simulink model "P4_sim_LQR"  (R2021b)
settings: Solver=ode45  StartTime=0.0  StopTime=Tmax  RelTol=1e-6  EnableMultiTasking=on
values from neighbouring files (symbols this model uses):
  a = g/L    (= 32.6666666667)    [P4_1.m]    (also in P4_2_1.m; P4_2_2.m; P4_2_3.m; P4_3.m)
  b = k/m    (= 0.1)    [P4_1.m]    (also in P4_2_1.m; P4_2_2.m; P4_2_3.m; P4_3.m)
  c = 1/(m*L^2)    (= 111.111111111)    [P4_1.m]    (also in P4_2_1.m; P4_2_2.m; P4_2_3.m; P4_3.m)
  du_max = 0.15    [P4_1.m]    (also in P4_2_1.m = 100; P4_2_2.m = 100; P4_2_3.m = du_vector(i); P4_3.m = 0.085)
  du_min = -0.15    [P4_1.m]    (also in P4_2_1.m = -100; P4_2_2.m = -100; P4_2_3.m = -du_vector(i); P4_3.m = -0.085)
  h = 0.1    [P4_1.m]    (also in P4_2_1.m; P4_2_2.m; P4_2_3.m; P4_3.m)
  KLQ = dlqr(Apd,Bpd,eye(2),R)    [P4_3.m]
  u_max = 0.15    [P4_1.m]    (also in P4_2_1.m = 100; P4_2_2.m = 100; P4_2_3.m = 100; P4_3.m = 0.22)
  u_min = -0.15    [P4_1.m]    (also in P4_2_1.m = -100; P4_2_2.m = -100; P4_2_3.m = -100; P4_3.m = -0.22)
settings Model: Creator=jomle  LastModifiedBy=User
settings SolverCC: AlgebraicLoopSolver=TrustRegion
settings DataIOCC: LimitDataPoints=on  SaveFormat=Array  ReturnWorkspaceOutputs=off
settings OptimizationCC: LifeSpan=inf
settings DebuggingCC: SFUnexpectedBacktrackingDiag=warning  SFNoUnconditionalDefaultTransitionDiag=warning  SFExecutionAtInitializationDiag=none  SFMachineParentedDataDiag=warning  ArithmeticOperatorsInVariantConditions=warning
settings HardwareCC: ProdBitPerPointer=32  ProdBitPerSizeT=32  ProdBitPerPtrDiffT=32  ProdLargestAtomicFloat=None  ProdIntDivRoundTo=Undefined  ProdEndianess=Unspecified  ProdWordSize=32  ProdHWDeviceType=32-bit Generic
settings ModelReferenceCC: PropagateSignalLabelsOutOfModel=off
settings SFSimCC: SimUseLocalCustomCode=off  CustomCodeUndefinedFunction=UseInterfaceOnly
settings RTWCC: RTWUseLocalCustomCode=off
settings CodeAppCC: StateflowObjectComments=on
settings GRTTargetCC: TargetLangStandard=C89/C90 (ANSI)
settings ConfigComp: CovMetricSettings=dw  CovSaveCumulativeToWorkspaceVar=on  CovSaveSingleToWorkspaceVar=on  CovExternalEMLEnable=off

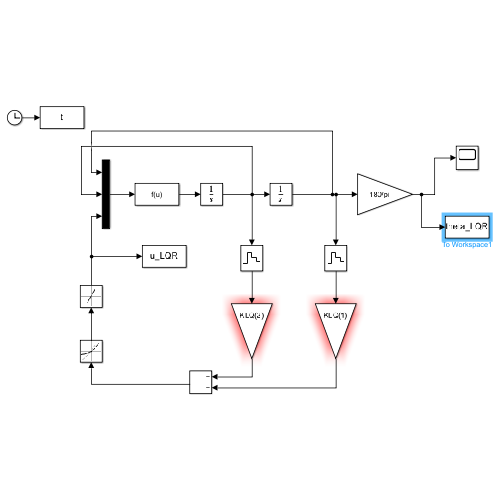
[thumbnail: Simulink's stored preview of the top-level diagram]
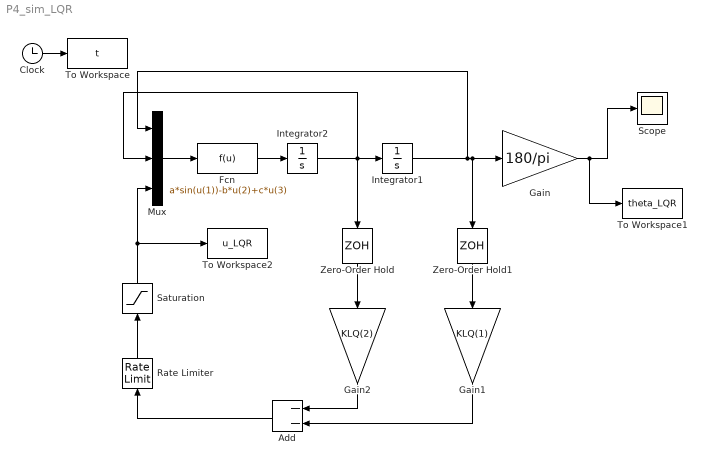
== system P4_sim_LQR ==
  Add : Sum  Inputs=--
  Clock : Clock
  Fcn : Fcn  Expr=a*sin(u(1))-b*u(2)+c*u(3)
  Gain : Gain  Gain=180/pi
  Gain1 : Gain  Gain=KLQ(1)
  Gain2 : Gain  Gain=KLQ(2)
  Integrator1 : Integrator  InitialCondition=30*pi/180
  Integrator2 : Integrator
  Mux : Mux  Inputs=3
  Rate Limiter : RateLimiter  RisingSlewLimit=du_max/h  FallingSlewLimit=du_min/h  SampleTimeMode=inherited
  Saturation : Saturate  UpperLimit=u_max  LowerLimit=u_min
  Scope : Scope
  To Workspace : ToWorkspace  VariableName=t  SampleTime=-1
  To Workspace1 : ToWorkspace  VariableName=theta_LQR  SampleTime=-1
  To Workspace2 : ToWorkspace  VariableName=u_LQR  SaveFormat=Structure With Time  SampleTime=-1
  Zero-Order Hold : ZeroOrderHold  SampleTime=h
  Zero-Order Hold1 : ZeroOrderHold  SampleTime=h
  wires:
  Integrator2/1 -> Mux/2, Zero-Order Hold/1, Integrator1/1
  Integrator1/1 -> Zero-Order Hold1/1, Gain/1, Mux/1
  Gain/1 -> To Workspace1/1, Scope/1
  Mux/1 -> Fcn/1
  Fcn/1 -> Integrator2/1
  Gain2/1 -> Add/1
  Gain1/1 -> Add/2
  Clock/1 -> To Workspace/1
  Zero-Order Hold/1 -> Gain2/1
  Zero-Order Hold1/1 -> Gain1/1
  Rate Limiter/1 -> Saturation/1
  Add/1 -> Rate Limiter/1
  Saturation/1 -> To Workspace2/1, Mux/3
